simulink library "AnnGainCalcBtc"  (R2022b)
settings: Solver=VariableStepAuto  StartTime=0.0  StopTime=10.0  RelTol=1e-3
libraries: TuneVar x5, FeaturePath x1, HandyTextFile x1, dspindex x1, dspmathops x1
settings Model: Creator=kl13806  LastModifiedBy=kl13806
settings SolverCC: AlgebraicLoopSolver=TrustRegion
settings DebuggingCC: UnconnectedInputMsg=warning  UnconnectedOutputMsg=warning  UnconnectedLineMsg=warning  SFMachineParentedDataDiag=warning
settings ModelReferenceCC: EnableRefExpFcnMdlSchedulingChecks=on
settings RTWCC: DLArmComputeVersion=19.05

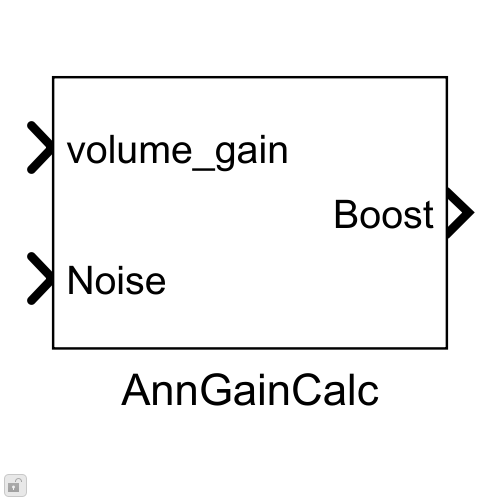
[thumbnail: Simulink's stored preview of the top-level diagram]
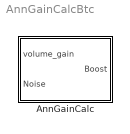
== system AnnGainCalcBtc ==
  AnnGainCalc : Subsystem  mask(Blocklib AnnGainCalc){Config=[], FeatureName=gaincalc}
      mask prompts: Config "AnnGainCalcConfig"; FeatureName "Feature path name:"
      mask init:
      | blkh=gcbh;
      | Config=BTConfig.Assert(blkh,Config);
      | %     rampWc      = 1/(Config.RampTau*Config.Fd);
      | %     rampSinCoef = sin(rampWc);
      | %     rampCosCoef = cos(rampWc);
      | %     Config.RampCoef    = (1-rampSinCoef)/rampCosCoef;  
      | Config.Validate();
      | BTConfig.InitSetFeatureIfPresent(blkh,'FeatureName');
      mask Callback Config: BTConfig.CallbackHideIfPresent(gcbh,{'FeatureName'});
      mask TypeOptions FeatureName: FeaturePath/FeatureName

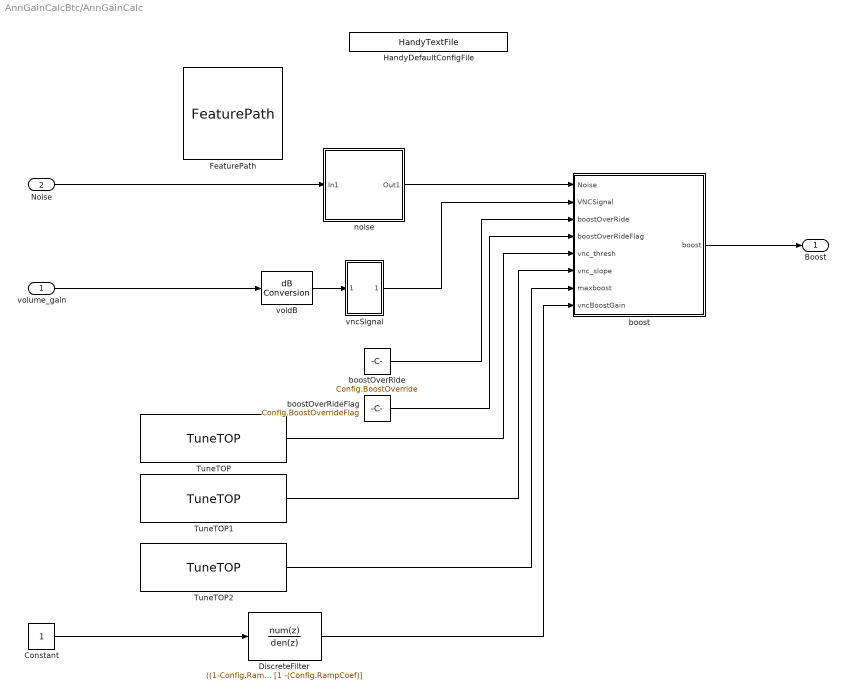
== system AnnGainCalcBtc/AnnGainCalc ==
  volume_gain : Inport
  Noise : Inport  Port=2
  Constant : Constant  OutDataTypeStr=single
  DiscreteFilter : DiscreteFilter  Numerator=((1-Config.RampCoef)*Config.VncEnable)  Denominator=[1 -(Config.RampCoef)]  InitialStates=Config.RampCoef*Config.VncBoostGain  InputProcessing=Columns as channels (frame based)  FilterStructure=Direct form II transposed  a0EqualsOne=on
  FeaturePath : FeaturePath/FeaturePath  FeatureName=gaincalc  IsGroup=off  GroupNumber=-1  IsModule=off  TriggerInit=[-350 -126 -235 -19]
      settings: SourceProductName=Bose Talaria
  HandyDefaultConfigFile : HandyTextFile/HandyTextFile  TemplateSource=Config  FileSuffix=Init  OpenDialogOnLoad=off  UseThisBlockName=off  AddGrandParentNamePrefix=off  TheDefaultText=|  ShowInLibBrowser=on
      | % $(FILENAME) Setup model parameters for each "Init" callback (e.g. update diagram)
      | sample_rate_in_hertz = 44100;
      | frame_size = 32;
      | sysin_channel_count = 2;
      settings: SourceProductName=Bose Talaria
  TuneTOP : TuneVar/TuneTOP  TriggerInit=[-400 277 -230 333]  TopName=VncThresh  TuneName=VncThresh  DataType=single  TunabilityNumber=1  MinValue=[]  MaxValue=[]  BankNumber=0  PreOverlay=false  PostOverlay=false  UseSameName=on  MaskValue=Config.VncThresh
      settings: SourceProductName=Bose Talaria
  TuneTOP1 : TuneVar/TuneTOP  TriggerInit=[-400 347 -230 403]  TopName=VncSlope  TuneName=VncSlope  DataType=single  TunabilityNumber=1  MinValue=[]  MaxValue=[]  BankNumber=0  PreOverlay=false  PostOverlay=false  UseSameName=on  MaskValue=Config.VncSlope
      settings: SourceProductName=Bose Talaria
  TuneTOP2 : TuneVar/TuneTOP  TriggerInit=[-400 427 -230 483]  TopName=MaxBoost  TuneName=MaxBoost  DataType=single  TunabilityNumber=1  MinValue=[]  MaxValue=[]  BankNumber=0  PreOverlay=false  PostOverlay=false  UseSameName=on  MaskValue=Config.MaxBoost
      settings: SourceProductName=Bose Talaria
  boost : Subsystem
  boostOverRide : Constant  Value=Config.BoostOverride  OutDataTypeStr=single
  boostOverRideFlag : Constant  Value=Config.BoostOverrideFlag  OutDataTypeStr=single
  noise : Subsystem
  vncSignal : Subsystem
  voldB : dspmathops/dB Conversion  dBtype=dB  intype=Amplitude  R=1  fuzz=on
  Boost : Outport  VectorParamsAs1DForOutWhenUnconnected=off
  wires:
  volume_gain/1 -> voldB/1
  Constant/1 -> DiscreteFilter/1
  vncSignal/1(Out1) -> boost/2(VNCSignal)
  voldB/1 -> vncSignal/1(In1)
  boostOverRide/1 -> boost/3(boostOverRide)
  boostOverRideFlag/1 -> boost/4(boostOverRideFlag)
  TuneTOP/1 -> boost/5(vnc_thresh)
  TuneTOP1/1 -> boost/6(vnc_slope)
  TuneTOP2/1 -> boost/7(maxboost)
  boost/1(boost) -> Boost/1
  DiscreteFilter/1 -> boost/8(vncBoostGain)
  Noise/1 -> noise/1(In1)
  noise/1(Out1) -> boost/1(Noise)

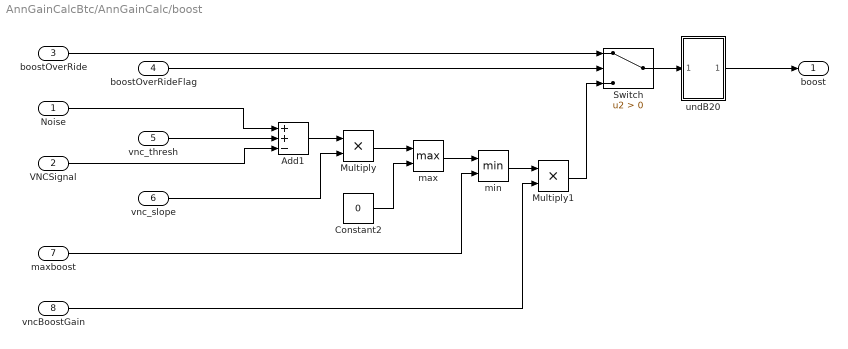
== system AnnGainCalcBtc/AnnGainCalc/boost ==
  Noise : Inport
  VNCSignal : Inport  Port=2
  boostOverRide : Inport  Port=3
  boostOverRideFlag : Inport  Port=4
  vnc_thresh : Inport  Port=5
  vnc_slope : Inport  Port=6
  maxboost : Inport  Port=7
  vncBoostGain : Inport  Port=8
  Add1 : Sum  Inputs=++-
  Constant2 : Constant  Value=0  OutDataTypeStr=single
  Multiply : Product
  Multiply1 : Product
  Switch : Switch  Criteria=u2 > Threshold  SaturateOnIntegerOverflow=off  InputSameDT=off
  max : MinMax  Function=max  Inputs=2
  min : MinMax  Inputs=2
  undB20 : Subsystem
  boost : Outport  VectorParamsAs1DForOutWhenUnconnected=off
  wires:
  boostOverRide/1 -> Switch/1
  Multiply1/1 -> Switch/3
  Add1/1 -> Multiply/1
  min/1 -> Multiply1/1
  VNCSignal/1 -> Add1/3
  max/1 -> min/1
  Noise/1 -> Add1/1
  Switch/1 -> undB20/1(In1)
  Constant2/1 -> max/2
  vnc_thresh/1 -> Add1/2
  Multiply/1 -> max/1
  boostOverRideFlag/1 -> Switch/2
  maxboost/1 -> min/2
  vncBoostGain/1 -> Multiply1/2
  vnc_slope/1 -> Multiply/2
  undB20/1(Out1) -> boost/1

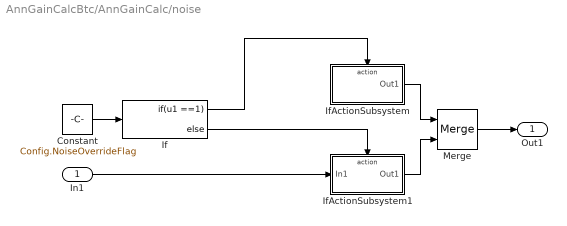
== system AnnGainCalcBtc/AnnGainCalc/noise ==
  In1 : Inport
  Constant : Constant  Value=Config.NoiseOverrideFlag  OutDataTypeStr=single
  If : If  IfExpression=u1 ==1
  IfActionSubsystem : Subsystem  TreatAsAtomicUnit=on
  IfActionSubsystem1 : Subsystem  TreatAsAtomicUnit=on
  Merge : Merge
  Out1 : Outport  VectorParamsAs1DForOutWhenUnconnected=off
  wires:
  If/2 -> IfActionSubsystem1/Action
  Constant/1 -> If/1
  IfActionSubsystem/1(Out1) -> Merge/1
  IfActionSubsystem1/1(Out1) -> Merge/2
  Merge/1 -> Out1/1
  If/1 -> IfActionSubsystem/Action
  In1/1 -> IfActionSubsystem1/1(In1)

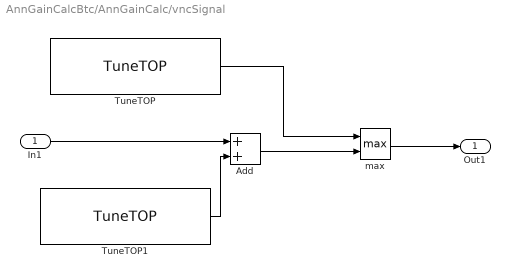
== system AnnGainCalcBtc/AnnGainCalc/vncSignal ==
  In1 : Inport
  Add : Sum
  TuneTOP : TuneVar/TuneTOP  TriggerInit=[50 -8 220 48]  TopName=MinVncSignal  TuneName=MinVncSignal  DataType=single  TunabilityNumber=1  MinValue=[]  MaxValue=[]  BankNumber=0  PreOverlay=false  PostOverlay=false  UseSameName=on  MaskValue=Config.MinVncSignal
      settings: SourceProductName=Bose Talaria
  TuneTOP1 : TuneVar/TuneTOP  TriggerInit=[40 142 210 198]  TopName=MaxSpl  TuneName=MaxSpl  DataType=single  TunabilityNumber=1  MinValue=[]  MaxValue=[]  BankNumber=0  PreOverlay=false  PostOverlay=false  UseSameName=on  MaskValue=Config.MaxSpl
      settings: SourceProductName=Bose Talaria
  max : MinMax  Function=max  Inputs=2
  Out1 : Outport  VectorParamsAs1DForOutWhenUnconnected=off
  wires:
  TuneTOP/1 -> max/1
  In1/1 -> Add/1
  Add/1 -> max/2
  TuneTOP1/1 -> Add/2
  max/1 -> Out1/1

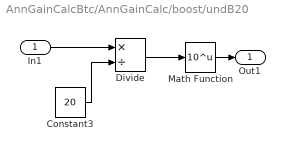
== system AnnGainCalcBtc/AnnGainCalc/boost/undB20 ==
  In1 : Inport
  Constant3 : Constant  Value=20  OutDataTypeStr=single
  Divide : Product  Inputs=*/
  Math Function : Math  Operator=10^u  SignedPower=on
  Out1 : Outport  VectorParamsAs1DForOutWhenUnconnected=off
  wires:
  Constant3/1 -> Divide/2
  Divide/1 -> Math Function/1
  Math Function/1 -> Out1/1
  In1/1 -> Divide/1

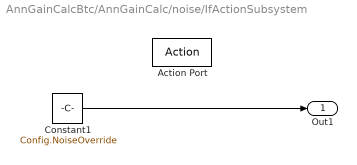
== system AnnGainCalcBtc/AnnGainCalc/noise/IfActionSubsystem ==
  Action Port : ActionPort
  Constant1 : Constant  Value=Config.NoiseOverride  OutDataTypeStr=single
  Out1 : Outport  VectorParamsAs1DForOutWhenUnconnected=off
  wires:
  Constant1/1 -> Out1/1

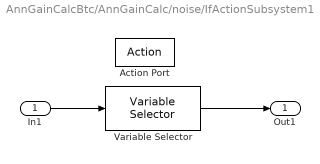
== system AnnGainCalcBtc/AnnGainCalc/noise/IfActionSubsystem1 ==
  In1 : Inport
  Action Port : ActionPort
  Variable Selector : dspindex/Variable Selector  NumInputs=1  rowsOrCols=Columns  IdxMode=Fixed  Elements=[1]  ZerOneIdxMode=One-based  errmode=Clip Index  FillMode=on  FillValues=0
  Out1 : Outport  OutDataTypeStr=single  VectorParamsAs1DForOutWhenUnconnected=off
  wires:
  In1/1 -> Variable Selector/1
  Variable Selector/1 -> Out1/1
